simulink model "Practica_control_ej_1_2_4"  (R2024b)
settings: Solver=VariableStepAuto  StartTime=0.0  StopTime=10.0  RelTol=1e-3
model workspace (MAT data in the model file):
  Jl = 5
  Jm = 0.25
  Kp = 500
  Kw = 50
  L = Simulink.Parameter
  L.Value = 0.05
  L.Complexity = 'real'
  L.Dimensions = [1 1]
  L.DataType = 'auto'
  R = 2
  n = 50
settings Model: Creator=Carlos  LastModifiedBy=Carlos

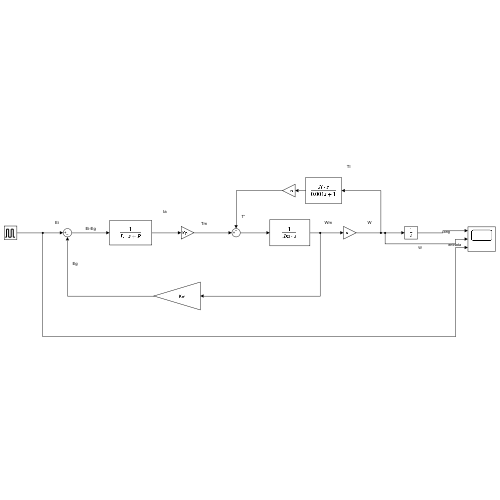
[thumbnail: Simulink's stored preview of the top-level diagram]
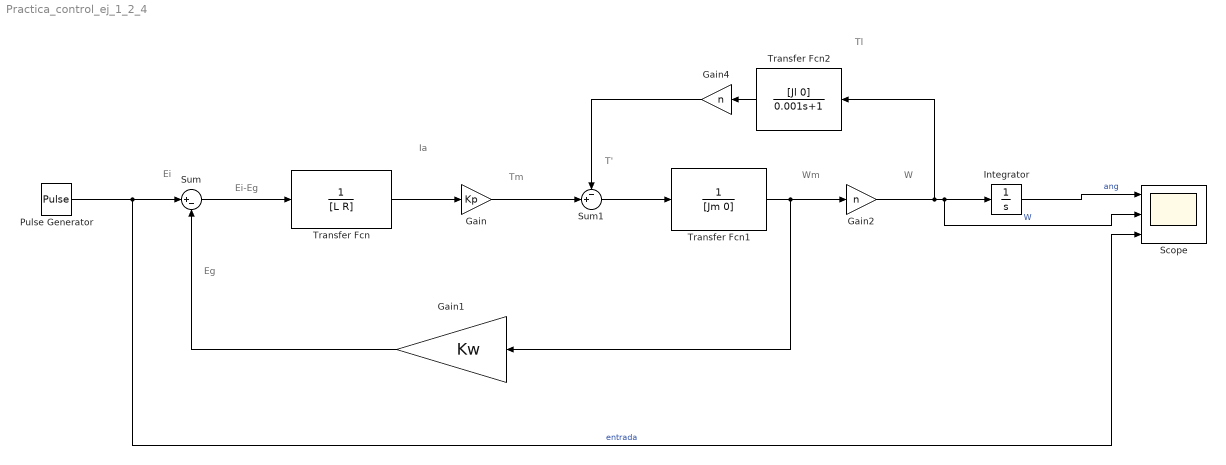
== system Practica_control_ej_1_2_4 ==
  note: Tl
  note: W
  note: Wm
  note: T'
  note: Tm
  note: Ia
  note: Ei-Eg
  note: Eg
  note: Ei
  Gain : Gain  Gain=Kp
  Gain1 : Gain  Gain=Kw
  Gain2 : Gain  Gain=n
  Gain4 : Gain  Gain=n
  Integrator : Integrator
  Pulse Generator : DiscretePulseGenerator  PulseType=Time based  Amplitude=100  PulseWidth=50
  Scope : Scope  NumInputPorts=3
  Sum : Sum  Inputs=|+-
  Sum1 : Sum  Inputs=-+|
  Transfer Fcn : TransferFcn  Denominator=[L R]
  Transfer Fcn1 : TransferFcn  Denominator=[Jm 0]
  Transfer Fcn2 : TransferFcn  Numerator=[Jl 0]  Denominator=[0.001 1]
  wires:
  Sum/1 -> Transfer Fcn/1
  Transfer Fcn/1 -> Gain/1
  Sum1/1 -> Transfer Fcn1/1
  Transfer Fcn1/1 -> Gain2/1, Gain1/1
  Gain1/1 -> Sum/2
  Gain/1 -> Sum1/2
  Transfer Fcn2/1 -> Gain4/1
  Gain4/1 -> Sum1/1
  Integrator/1 -> Scope/1  "ang"
  Gain2/1 -> Transfer Fcn2/1, Scope/2, Integrator/1  "W"
  Pulse Generator/1 -> Scope/3, Sum/1  "entrada"
